simulink model "BusSelector5"  (R2017b)
settings: Solver=FixedStepAuto  StartTime=0.0  StopTime=10.0  FixedStep=0.200000  RelTol=1e-3
settings Model: Creator=hbourbou  LastModifiedBy=hbourbou

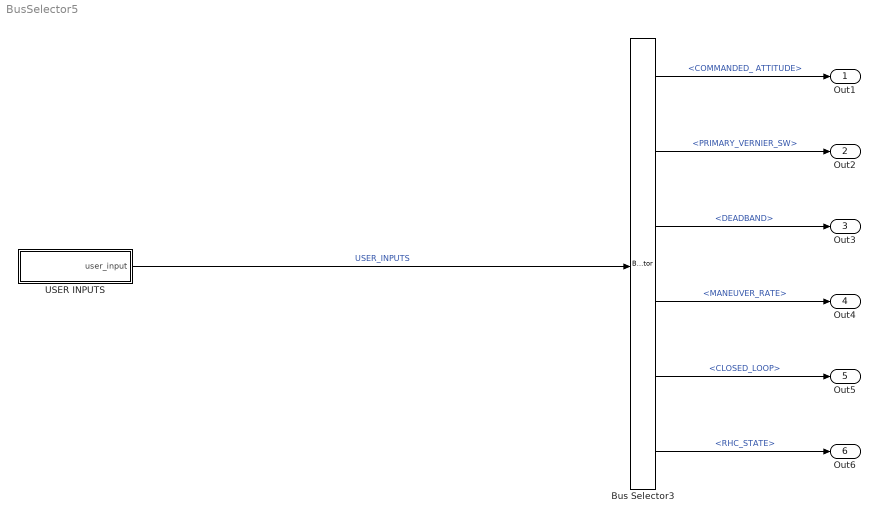
== system BusSelector5 ==
  Bus Selector3 : BusSelector  OutputSignals=COMMANDED_ ATTITUDE,PRIMARY_VERNIER_SW,DEADBAND,MANEUVER_RATE,CLOSED_LOOP,RHC_STATE
  USER INPUTS : Subsystem  Priority=1
  Out1 : Outport
  Out2 : Outport  Port=2
  Out3 : Outport  Port=3
  Out4 : Outport  Port=4
  Out5 : Outport  Port=5
  Out6 : Outport  Port=6
  wires:
  USER INPUTS/1(user_input) -> Bus Selector3/1  "USER_INPUTS"
  Bus Selector3/1 -> Out1/1  "<COMMANDED_ ATTITUDE>"
  Bus Selector3/2 -> Out2/1  "<PRIMARY_VERNIER_SW>"
  Bus Selector3/3 -> Out3/1  "<DEADBAND>"
  Bus Selector3/4 -> Out4/1  "<MANEUVER_RATE>"
  Bus Selector3/5 -> Out5/1  "<CLOSED_LOOP>"
  Bus Selector3/6 -> Out6/1  "<RHC_STATE>"

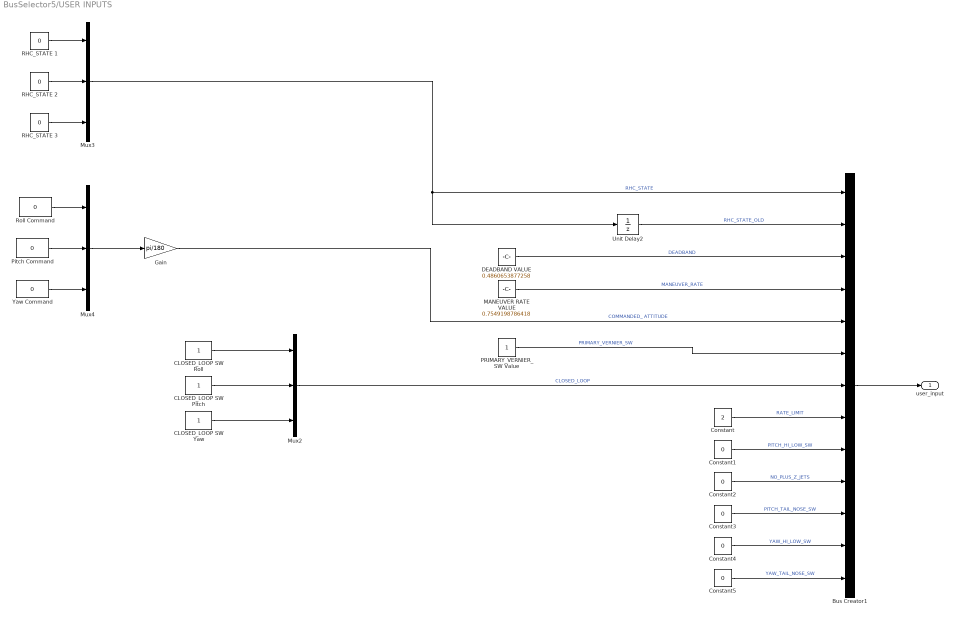
== system BusSelector5/USER INPUTS ==
  Bus Creator1 : BusCreator  Inputs=13
  CLOSED_LOOP SW Pitch : Constant  OutDataTypeStr=boolean
  CLOSED_LOOP SW Roll : Constant  OutDataTypeStr=boolean
  CLOSED_LOOP SW Yaw : Constant  OutDataTypeStr=boolean
  Constant : Constant  Value=2
  Constant{1..5} (5 alike) : Constant  Value=0  OutDataTypeStr=boolean
  DEADBAND VALUE : Constant  Value=0.4860653877258
  Gain : Gain  Gain=pi/180
  MANEUVER RATE VALUE : Constant  Value=0.7549198786418
  Mux2 : Mux  Inputs=3
  Mux3 : Mux  Inputs=3
  Mux4 : Mux  Inputs=3
  PRIMARY_VERNIER_SW Value : Constant
  Pitch Command : Constant  Value=0
  RHC_STATE 1 : Constant  Value=0  OutDataTypeStr=int8
  RHC_STATE 2 : Constant  Value=0  OutDataTypeStr=int8
  RHC_STATE 3 : Constant  Value=0  OutDataTypeStr=int8
  Roll Command : Constant  Value=0
  Unit Delay2 : UnitDelay  SampleTime=-1
  Yaw Command : Constant  Value=0
  user_input : Outport
  wires:
  RHC_STATE 1/1 -> Mux3/1
  RHC_STATE 3/1 -> Mux3/3
  DEADBAND VALUE/1 -> Bus Creator1/3  "DEADBAND"
  MANEUVER RATE VALUE/1 -> Bus Creator1/4  "MANEUVER_RATE"
  Gain/1 -> Bus Creator1/5  "COMMANDED_ ATTITUDE"
  Mux2/1 -> Bus Creator1/7  "CLOSED_LOOP"
  CLOSED_LOOP SW Roll/1 -> Mux2/1
  CLOSED_LOOP SW Pitch/1 -> Mux2/2
  CLOSED_LOOP SW Yaw/1 -> Mux2/3
  RHC_STATE 2/1 -> Mux3/2
  Constant/1 -> Bus Creator1/8  "RATE_LIMIT"
  Constant1/1 -> Bus Creator1/9  "PITCH_HI_LOW_SW"
  Constant2/1 -> Bus Creator1/10  "NO_PLUS_Z_JETS"
  Constant3/1 -> Bus Creator1/11  "PITCH_TAIL_NOSE_SW"
  Constant4/1 -> Bus Creator1/12  "YAW_HI_LOW_SW"
  Constant5/1 -> Bus Creator1/13  "YAW_TAIL_NOSE_SW"
  Mux3/1 -> Unit Delay2/1, Bus Creator1/1  "RHC_STATE"
  Yaw Command/1 -> Mux4/3
  Pitch Command/1 -> Mux4/2
  Roll Command/1 -> Mux4/1
  Mux4/1 -> Gain/1
  PRIMARY_VERNIER_SW Value/1 -> Bus Creator1/6  "PRIMARY_VERNIER_SW"
  Unit Delay2/1 -> Bus Creator1/2  "RHC_STATE_OLD"
  Bus Creator1/1 -> user_input/1
